simulink model "MotionPlanner"  (R2020b)
settings: Solver=FixedStepAuto  StartTime=0.0  StopTime=10.0  FixedStep=Ts  MaxStep=0.02  RelTol=1e-3
values from neighbouring files (symbols this model uses):
  Ts = 0.1    [setupscript.m]
undefined symbols (not defined in the file or in its folder): DiscIntNeverNeededParam, globalPlanPoints
libraries: simulink x1
settings Model: Creator=The MathWorks, Inc.  LastModifiedBy=The MathWorks, Inc.
settings OptimizationCC: DefaultParameterBehavior=Inlined  EnhancedBackFolding=on  PassReuseOutputArgsAs=Individual arguments  ZeroExternalMemoryAtStartup=off  ZeroInternalMemoryAtStartup=off  OptimizeBlockOrder=speed  DifferentSizesBufferReuse=on  OptimizationCustomize=off  EfficientTunableParamExpr=on
settings DebuggingCC: ParameterTunabilityLossMsg=error  ModelReferenceSymbolNameMessage=none
settings ModelReferenceCC: ModelReferenceNumInstancesAllowed=Single  PropagateVarSize=During execution
settings SFSimCC: MATLABDynamicMemAllocThreshold=0
settings RTWCC: Description=Embedded Coder  SystemTargetFile=ert.tlc  TemplateMakefile=ert_default_tmf
settings CodeAppCC: ForceParamTrailComments=on  IgnoreCustomStorageClasses=off  OperatorAnnotations=on  SimulinkDataObjDesc=on  SFDataObjDesc=on  InsertBlockDesc=on
settings ERTTargetCC: TargetLangStandard=C99 (ISO)  GenerateSampleERTMain=on  SupportVariableSizeSignals=on  InlinedParameterPlacement=NonHierarchical  ERTCustomFileTemplate=example_file_process.tlc

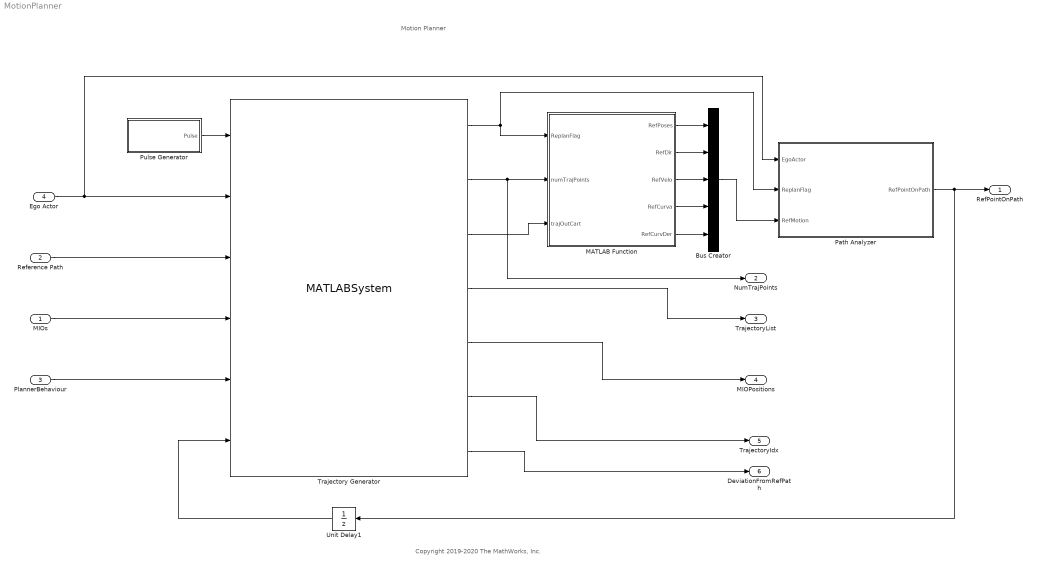
== system MotionPlanner ==
  note: Motion Planner
  note: Copyright 2019-2020 The MathWorks, Inc.
  MIOs : Inport  OutDataTypeStr=Bus: BusMIOs  BusOutputAsStruct=on
  Reference Path : Inport  Port=2  OutDataTypeStr=double  PortDimensions=size(globalPlanPoints)  Interpolate=off
  PlannerBehaviour : Inport  Port=3  OutDataTypeStr=Bus: BusPlannerBehavior  BusOutputAsStruct=on
  Ego Actor : Inport  Port=4  OutDataTypeStr=Bus: BusActors1Actors  Unit=m  BusOutputAsStruct=on
  Bus Creator : BusCreator  Inputs=5
  MATLAB Function : MATLAB Function  TreatAsAtomicUnit=on
  Path Analyzer : Subsystem  TreatAsAtomicUnit=on
  Pulse Generator : Subsystem  mask(Pulse Generator){pulsePeriod=1, sampleTime=0.1}
      mask prompts: pulsePeriod "Pulse period (sec)"; sampleTime "Sample time (sec)"
      mask help: Generates a periodic pulse. The pulse is high for the first sample of the period and then is low for the remained of the period.
  Trajectory Generator : MATLABSystem  System=HelperTrajectoryGenerator  SimulateUsing=Interpreted execution
      mask Type: HelperTrajectoryGenerator
      mask Display:
      | disp('HelperTrajectoryGenerator');
      | port_label('input',1,'ReplanFlag');
      | port_label('input',2,'EgoActor');
      | port_label('input',3,'RefPath');
      | port_label('input',4,'MIOs');
      | port_label('input',5,'PlannerBehavior');
      | port_label('input',6,'RefPointOnPath');
      | port_label('output',1,'isTrajNew');
      | port_label('output',2,'NumTrajPoints');
      | port_label('output',3,'Trajectory');
      | port_label('output',4,'TrajectoryList');
      | port_label('output',5,'MioPositions');
      | port_label('output',6,'TrajectoryIdx');
      | port_label('output',7,'LateralDeviation');
  Unit Delay1 : UnitDelay  SampleTime=-1  HasFrameUpgradeWarning=on
  RefPointOnPath : Outport  OutDataTypeStr=Bus: BusRefPointOnPath  VectorParamsAs1DForOutWhenUnconnected=off  BusOutputAsStruct=on
  NumTrajPoints : Outport  Port=2  Unit=m  VectorParamsAs1DForOutWhenUnconnected=off
  TrajectoryList : Outport  Port=3
  MIOPositions : Outport  Port=4
  TrajectoryIdx : Outport  Port=5
  DeviationFromRefPath : Outport  Port=6
  wires:
  Reference Path/1 -> Trajectory Generator/3
  MATLAB Function/2(RefDir) -> Bus Creator/2
  Trajectory Generator/1 -> MATLAB Function/1(ReplanFlag), Path Analyzer/2(ReplanFlag)
  MIOs/1 -> Trajectory Generator/4
  PlannerBehaviour/1 -> Trajectory Generator/5
  Bus Creator/1 -> Path Analyzer/3(RefMotion)
  MATLAB Function/5(RefCurvDer) -> Bus Creator/5
  Path Analyzer/1(RefPointOnPath) -> Unit Delay1/1, RefPointOnPath/1
  MATLAB Function/3(RefVelo) -> Bus Creator/3
  Trajectory Generator/5 -> MIOPositions/1
  MATLAB Function/1(RefPoses) -> Bus Creator/1
  Ego Actor/1 -> Path Analyzer/1(EgoActor), Trajectory Generator/2
  Trajectory Generator/4 -> TrajectoryList/1
  Trajectory Generator/2 -> NumTrajPoints/1, MATLAB Function/2(numTrajPoints)
  Pulse Generator/1(Pulse) -> Trajectory Generator/1
  MATLAB Function/4(RefCurva) -> Bus Creator/4
  Trajectory Generator/3 -> MATLAB Function/3(trajOutCart)
  Unit Delay1/1 -> Trajectory Generator/6
  Trajectory Generator/6 -> TrajectoryIdx/1
  Trajectory Generator/7 -> DeviationFromRefPath/1

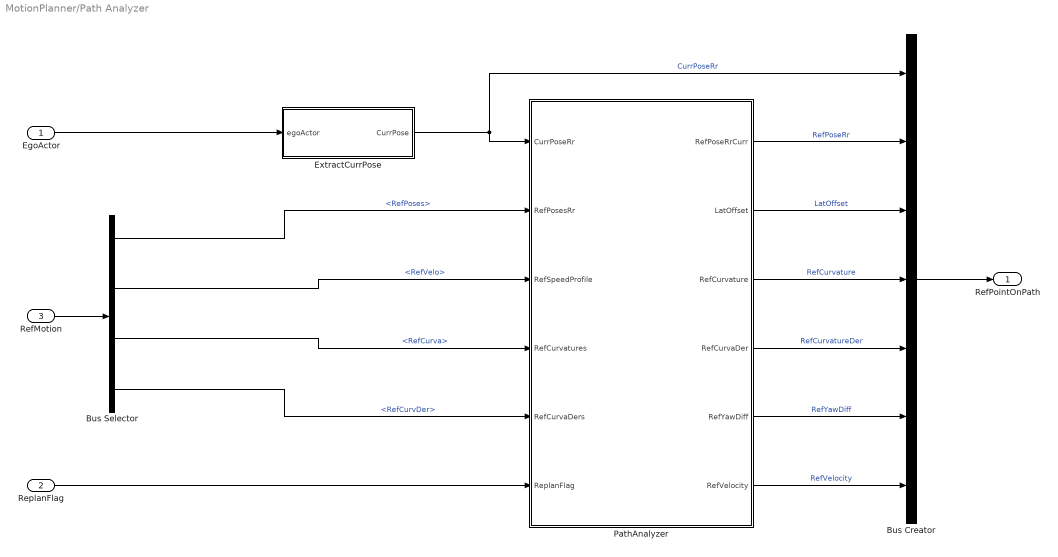
== system MotionPlanner/Path Analyzer ==
  EgoActor : Inport
  ReplanFlag : Inport  Port=2
  RefMotion : Inport  Port=3
  Bus Creator : BusCreator  Inputs=7  OutDataTypeStr=Bus: BusRefPointOnPath  NonVirtualBus=on
  Bus Selector : BusSelector  OutputSignals=RefPoses,RefVelo,RefCurva,RefCurvDer
  ExtractCurrPose : MATLAB Function  TreatAsAtomicUnit=on
  PathAnalyzer : Subsystem  TreatAsAtomicUnit=on
      settings: RTWFcnNameOpts=Use subsystem name
  RefPointOnPath : Outport  OutDataTypeStr=Bus: BusRefPointOnPath
  wires:
  ExtractCurrPose/1(CurrPose) -> Bus Creator/1, PathAnalyzer/1(CurrPoseRr)  "CurrPoseRr"
  PathAnalyzer/1(RefPoseRrCurr) -> Bus Creator/2  "RefPoseRr"
  EgoActor/1 -> ExtractCurrPose/1(egoActor)
  PathAnalyzer/4(RefCurvaDer) -> Bus Creator/5  "RefCurvatureDer"
  PathAnalyzer/3(RefCurvature) -> Bus Creator/4  "RefCurvature"
  PathAnalyzer/5(RefYawDiff) -> Bus Creator/6  "RefYawDiff"
  PathAnalyzer/2(LatOffset) -> Bus Creator/3  "LatOffset"
  Bus Creator/1 -> RefPointOnPath/1
  PathAnalyzer/6(RefVelocity) -> Bus Creator/7  "RefVelocity"
  RefMotion/1 -> Bus Selector/1
  Bus Selector/1 -> PathAnalyzer/2(RefPosesRr)  "<RefPoses>"
  Bus Selector/2 -> PathAnalyzer/3(RefSpeedProfile)  "<RefVelo>"
  Bus Selector/3 -> PathAnalyzer/4(RefCurvatures)  "<RefCurva>"
  Bus Selector/4 -> PathAnalyzer/5(RefCurvaDers)  "<RefCurvDer>"
  ReplanFlag/1 -> PathAnalyzer/6(ReplanFlag)

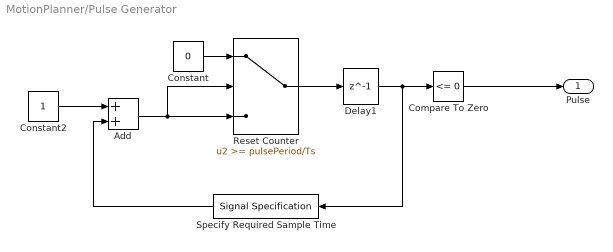
== system MotionPlanner/Pulse Generator ==
  Add : Sum
  Compare To Zero : simulink/Logic and Bit Operations/Compare To Zero  relop=<=  OutDataTypeStr=boolean
  Constant : Constant  Value=0
  Constant2 : Constant
  Delay1 : Delay  DelayLength=1
  Reset Counter : Switch  Threshold=pulsePeriod/Ts
      settings: AttributesFormatString=|
      | ----------------------------
      | Threshold = %<Threshold>
  Specify Required Sample Time : SignalSpecification  SampleTime=sampleTime
  Pulse : Outport
  wires:
  Reset Counter/1 -> Delay1/1
  Add/1 -> Reset Counter/3, Reset Counter/2
  Specify Required Sample Time/1 -> Add/2
  Delay1/1 -> Specify Required Sample Time/1, Compare To Zero/1
  Constant2/1 -> Add/1
  Constant/1 -> Reset Counter/1
  Compare To Zero/1 -> Pulse/1

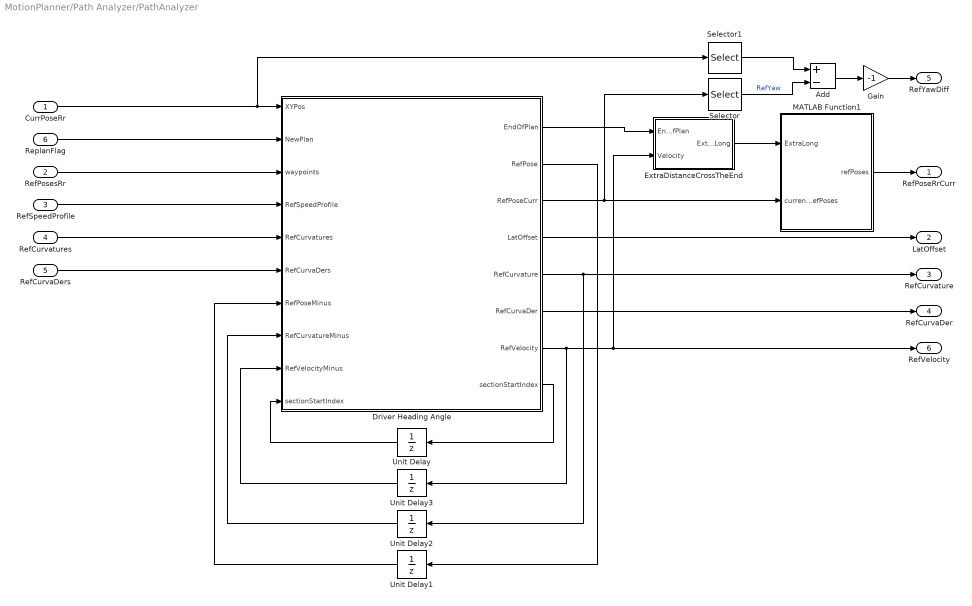
== system MotionPlanner/Path Analyzer/PathAnalyzer ==
  CurrPoseRr : Inport
  RefPosesRr : Inport  Port=2
  RefSpeedProfile : Inport  Port=3
  RefCurvatures : Inport  Port=4
  RefCurvaDers : Inport  Port=5
  ReplanFlag : Inport  Port=6
  Add : Sum  Inputs=+-
  Driver Heading Angle : MATLAB Function  TreatAsAtomicUnit=on
  ExtraDistanceCrossTheEnd : Subsystem
  Gain : Gain  Gain=-1
  MATLAB Function1 : MATLAB Function  TreatAsAtomicUnit=on
  Selector : Selector  InputPortWidth=3  IndexOptions=Index vector (dialog)  Indices=[3]  OutputSizes=1
  Selector1 : Selector  InputPortWidth=3  IndexOptions=Index vector (dialog)  Indices=[3]  OutputSizes=1
  Unit Delay : UnitDelay  SampleTime=-1  HasFrameUpgradeWarning=on
  Unit Delay1 : UnitDelay  InitialCondition=[0 0 0]  SampleTime=-1  HasFrameUpgradeWarning=on
  Unit Delay2 : UnitDelay  SampleTime=-1  HasFrameUpgradeWarning=on
  Unit Delay3 : UnitDelay  SampleTime=-1  HasFrameUpgradeWarning=on
  RefPoseRrCurr : Outport  VectorParamsAs1DForOutWhenUnconnected=off
  LatOffset : Outport  Port=2  VectorParamsAs1DForOutWhenUnconnected=off
  RefCurvature : Outport  Port=3  VectorParamsAs1DForOutWhenUnconnected=off
  RefCurvaDer : Outport  Port=4  VectorParamsAs1DForOutWhenUnconnected=off
  RefYawDiff : Outport  Port=5  VectorParamsAs1DForOutWhenUnconnected=off
  RefVelocity : Outport  Port=6  VectorParamsAs1DForOutWhenUnconnected=off
  wires:
  Unit Delay/1 -> Driver Heading Angle/10("sectionStartIndex ")
  Unit Delay1/1 -> Driver Heading Angle/7(RefPoseMinus)
  CurrPoseRr/1 -> Driver Heading Angle/1(XYPos), Selector1/1
  RefPosesRr/1 -> Driver Heading Angle/3(waypoints)
  RefSpeedProfile/1 -> Driver Heading Angle/4(RefSpeedProfile)
  Driver Heading Angle/7(RefVelocity) -> ExtraDistanceCrossTheEnd/2(Velocity), RefVelocity/1, Unit Delay3/1
  Driver Heading Angle/1(EndOfPlan) -> ExtraDistanceCrossTheEnd/1(EndOfPlan)
  Driver Heading Angle/3(RefPoseCurr) -> Selector/1, MATLAB Function1/2(currentRefPoses)
  RefCurvatures/1 -> Driver Heading Angle/5(RefCurvatures)
  Driver Heading Angle/8(sectionStartIndex) -> Unit Delay/1
  Driver Heading Angle/5(RefCurvature) -> RefCurvature/1, Unit Delay2/1
  Unit Delay2/1 -> Driver Heading Angle/8(RefCurvatureMinus)
  Unit Delay3/1 -> Driver Heading Angle/9(RefVelocityMinus)
  Driver Heading Angle/2(RefPose) -> Unit Delay1/1
  Add/1 -> Gain/1
  Selector1/1 -> Add/1
  Selector/1 -> Add/2  "RefYaw"
  ExtraDistanceCrossTheEnd/1(ExtraLong) -> MATLAB Function1/1(ExtraLong)
  MATLAB Function1/1(refPoses) -> RefPoseRrCurr/1
  Gain/1 -> RefYawDiff/1
  RefCurvaDers/1 -> Driver Heading Angle/6(RefCurvaDers)
  Driver Heading Angle/6(RefCurvaDer) -> RefCurvaDer/1
  Driver Heading Angle/4(LatOffset) -> LatOffset/1
  ReplanFlag/1 -> Driver Heading Angle/2(NewPlan)

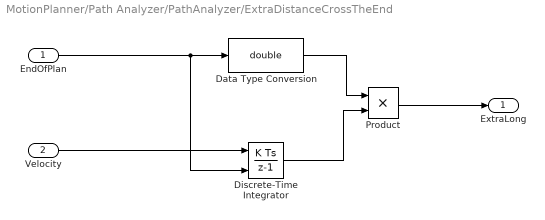
== system MotionPlanner/Path Analyzer/PathAnalyzer/ExtraDistanceCrossTheEnd ==
  EndOfPlan : Inport
  Velocity : Inport  Port=2
  Data Type Conversion : DataTypeConversion  OutDataTypeStr=double
  Discrete-Time Integrator : DiscreteIntegrator  ExternalReset=rising  SampleTime=-1  ICPrevOutput=DiscIntNeverNeededParam  ICPrevScaledInput=DiscIntNeverNeededParam
  Product : Product
  ExtraLong : Outport  VectorParamsAs1DForOutWhenUnconnected=off
  wires:
  Product/1 -> ExtraLong/1
  Data Type Conversion/1 -> Product/1
  Velocity/1 -> Discrete-Time Integrator/1
  Discrete-Time Integrator/1 -> Product/2
  EndOfPlan/1 -> Data Type Conversion/1, Discrete-Time Integrator/2

== matlab function MotionPlanner/Path Analyzer/ExtractCurrPose ==
  data: egoActor input; CurrPose output
%% getEgoPose
% Extracts ego position form the bus
function CurrPose = getEgoPose(egoActor)
    CurrPose = [egoActor.Position(1:2) egoActor.Yaw];
end

== matlab function MotionPlanner/MATLAB Function ==
  data: ReplanFlag input; RefPoses output; numTrajPoints input; trajOutCart input; RefDir output; RefVelo output; RefCurva output; RefCurvDer output
function [RefPoses,RefDir,RefVelo,RefCurva,RefCurvDer]  = extractStates(ReplanFlag,...
                                                          numTrajPoints, trajOutCart)
% This function parses the Trajectory generated by planner:
% Trajectory generated by the planner is extracted to get Position, 
% Curvature, Velocity, Curvature Derivative.
persistent RefPosesState RefVeloState RefCurvaState RefCurvaDerState

% Initialize the persistent variables 
if isempty(RefPosesState)
    RefPosesState = zeros(500,3);
    RefVeloState  = zeros(500,1);
    RefCurvaState = zeros(500,1);
    RefCurvaDerState = zeros(500,1);
end

% Chek for the new trajectory
% Parse the cartesian states of trajectory (trajOutCart)
if ReplanFlag
    TimeVecInTraj = trajOutCart(1:numTrajPoints,7);    
    TimeVecResample = linspace(TimeVecInTraj(1),TimeVecInTraj(end),500)';
    RefPosesState(:,1) = interp1(TimeVecInTraj,trajOutCart(1:numTrajPoints,1),TimeVecResample);
    RefPosesState(:,2) = interp1(TimeVecInTraj,trajOutCart(1:numTrajPoints,2),TimeVecResample);
    RefPosesState(:,3) = interp1(TimeVecInTraj,trajOutCart(1:numTrajPoints,3),TimeVecResample)/pi*180;
    RefVeloState       = interp1(TimeVecInTraj,trajOutCart(1:numTrajPoints,5),TimeVecResample);
    RefCurvaState      = interp1(TimeVecInTraj,trajOutCart(1:numTrajPoints,4),TimeVecResample);
    RefCurvaDerState    = gradient(RefCurvaState)./gradient(TimeVecResample)./RefVeloState;
end

% Assign the values to output variables
RefPoses = RefPosesState;
RefDir   = ones(500,1);
RefVelo  = RefVeloState;
RefCurva = RefCurvaState;
RefCurvDer = RefCurvaDerState;
end

== matlab function MotionPlanner/Path Analyzer/PathAnalyzer/Driver Heading Angle ==
  data: XYPos input; NewPlan input; EndOfPlan output boolean size=1; RefPose output double size=[1 3]; RefPoseCurr output double size=[1 3]; LatOffset output; RefCurvature output double size=1; RefCurvaDer output; RefVelocity output double; waypoints input; RefSpeedProfile input; RefCurvatures input; RefCurvaDers input; RefPoseMinus input size=[1 3]; RefCurvatureMinus input; RefVelocityMinus input; sectionStartIndex input double size=1; sectionStartIndex output
%% exampleHelperDriverHadingCalculator
% This function calculates the next best point from the trajectory
% The output of this block will be used to calculatethe inputs for path
% following controller
function [EndOfPlan,RefPose,RefPoseCurr,LatOffset,RefCurvature,RefCurvaDer,RefVelocity,sectionStartIndex] = exampleHelperDriverHadingCalculator(XYPos, NewPlan,waypoints, RefSpeedProfile, RefCurvatures, RefCurvaDers, RefPoseMinus, RefCurvatureMinus, RefVelocityMinus, sectionStartIndex)
% DRIVERHEADINGANGLE
% XYPos     = Current position of vehicle
% waypoints = Desired path
% phid      = Desired heading angle
if NewPlan
    sectionStartIndex = 1;
end

if sectionStartIndex < 1
    sectionStartIndex = 1;
end

EndOfPlan    = false;
RefPose      = zeros(1, 3);
RefPoseCurr  = zeros(1, 3);
RefCurvature = 0;
RefVelocity  = 1;


numWaypoints = size(waypoints,1);
if (numWaypoints == 0)
    return;
end

% Distance between section start and end points
DeltaXY = [waypoints(sectionStartIndex+1,1)-waypoints(sectionStartIndex,1),...
           waypoints(sectionStartIndex+1,2)-waypoints(sectionStartIndex,2)];

% Distance between current position and section starting point
RXY = [XYPos(1)-waypoints(sectionStartIndex,1),...
       XYPos(2)-waypoints(sectionStartIndex,2)];

% Normalized distance between current position and section starting point
u = (RXY.*DeltaXY)/(DeltaXY.*DeltaXY);

% Find section ending point
indexIncrement = ceil(u-1);

if indexIncrement<0
    % In current section
    indexIncrement = 0;
end
if u >=1
    % Increment to appropriate section 
    % with the assumption that the distance between waypoints is 
    % approximately equal for near sections
    sectionStartIndex = sectionStartIndex+indexIncrement;
    % Adjust u to account for new section starting point
    u = u - indexIncrement;
end

if sectionStartIndex < (numWaypoints-1)
    % Operating within valid sections
    currentSectionEndIndex = sectionStartIndex+1;
    nextSectionEndIndex    = currentSectionEndIndex+1;
    % Target States at end point of current and next sections
    XYTarget0 = [waypoints(sectionStartIndex,1),...
                 waypoints(sectionStartIndex,2)];
    XYTarget1 = [waypoints(currentSectionEndIndex,1),...
                 waypoints(currentSectionEndIndex,2)];
    XYTarget2 = [waypoints(nextSectionEndIndex,1),...
                 waypoints(nextSectionEndIndex,2)];
    YawTarget0 = waypoints(sectionStartIndex,3);
    YawTarget1 = waypoints(currentSectionEndIndex,3);
    YawTarget2 = waypoints(nextSectionEndIndex,3);
    
    VelocityTarget1 = RefSpeedProfile(currentSectionEndIndex);
    VelocityTarget2 = RefSpeedProfile(nextSectionEndIndex);
    
    CurvatureTarget1 = RefCurvatures(currentSectionEndIndex);
    CurvatureTarget2 = RefCurvatures(nextSectionEndIndex);
    
    CurvaDerTarget1 = RefCurvaDers(currentSectionEndIndex);
    CurvaDerTarget2 = RefCurvaDers(nextSectionEndIndex);
    % Section weights         
    Weight1 = (1-u);
    Weight2 = u;
    % Target position
    XYTargetCurr = Weight1*XYTarget0+Weight2*XYTarget1;
    YawTargetCurr = Weight1*YawTarget0+Weight2*YawTarget1;
    XYTarget = Weight1*XYTarget1+Weight2*XYTarget2;
    YawTarget = Weight1*YawTarget1+Weight2*YawTarget2;
    % Desired RefPose
    RefPoseCurr = [XYTargetCurr YawTargetCurr];
    RefPose = [XYTarget YawTarget];
    % Desired velocity
    RefVelocity = Weight1*VelocityTarget1+Weight2*VelocityTarget2;
    % Desired curvature
    RefCurvature = Weight1*CurvatureTarget1+Weight2*CurvatureTarget2;
    RefCurvaDer = Weight1*CurvaDerTarget1+Weight2*CurvaDerTarget2;
    EndOfPlan = false;
else
    % Maintain last heading between points
    RefPoseCurr = RefPoseMinus;
    RefPose = RefPoseMinus;
    RefVelocity = RefVelocityMinus;
    RefCurvature = RefCurvatureMinus;
    RefCurvaDer  = 0;
    sectionStartIndex = numWaypoints-1;
    EndOfPlan = true;
end

% Distance between current position and RefPosCurr
Dist2Ref = [XYPos(1)-RefPoseCurr(1),...
       XYPos(2)-RefPoseCurr(2)];

% DirSign = DirectionOfPoint(waypoints(sectionStartIndex,1:2),waypoints(sectionStartIndex+1,1:2),RefPoseCurr);
DirSign = sign(CrossProd(DeltaXY(1),DeltaXY(2),Dist2Ref(1),Dist2Ref(2)));
LatOffset = -sqrt(Dist2Ref(1)^2+Dist2Ref(2)^2)*DirSign;
end

%%CrossProd Computes cross product of two vectors.
function CP = CrossProd(x1,y1,x2,y2)
CP = x1*y2-y1*x2;
end

== matlab function MotionPlanner/Path Analyzer/PathAnalyzer/MATLAB Function1 ==
  data: ExtraLong input; currentRefPoses input; refPoses output
%% extrapolateRefPoses
% Extrapolates the ref position from the trajectory for smooth motion
function refPoses = extrapolateRefPoses(ExtraLong, currentRefPoses)

refPoses = currentRefPoses+[ExtraLong 0 0;];
end
